simulink model "nonlinear_ode_model"  (R2024a)
settings: Solver=ode45  StartTime=2.0  StopTime=5.0  MaxStep=0.01  RelTol=1e-3
libraries: simulink x1
settings Model: Creator=andrey  LastModifiedBy=andrey

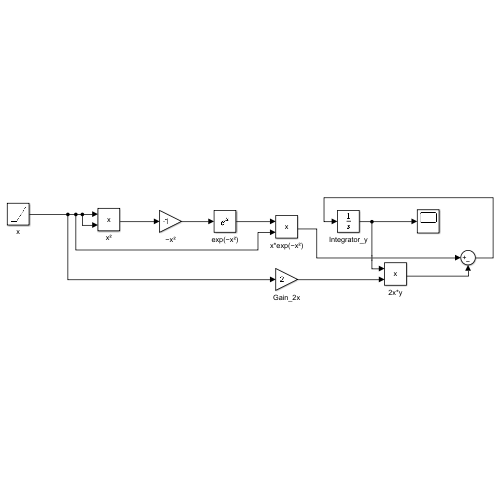
[thumbnail: Simulink's stored preview of the top-level diagram]
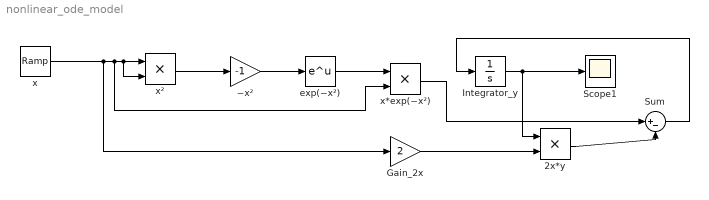
== system nonlinear_ode_model ==
  2x*y : Product
  Gain_2x : Gain  Gain=2
  Integrator_y : Integrator  InitialCondition=2
  Scope1 : Scope
  Sum : Sum  Inputs=|+-
  exp(−x²) : Math
  x : simulink/Sources/Ramp  slope=1  start=0  InitialOutput=0
  x*exp(−x²) : Product
  x² : Product
  −x² : Gain  Gain=-1
  wires:
  Integrator_y/1 -> 2x*y/1, Scope1/1
  x/1 -> Gain_2x/1, x*exp(−x²)/2, x²/2, x²/1
  x²/1 -> −x²/1
  −x²/1 -> exp(−x²)/1
  exp(−x²)/1 -> x*exp(−x²)/1
  Gain_2x/1 -> 2x*y/2
  x*exp(−x²)/1 -> Sum/1
  2x*y/1 -> Sum/2
  Sum/1 -> Integrator_y/1
